simulink model "BLOQUEPSK"  (Simulink 8.4)
settings: Solver=ode45  StartTime=0.0  StopTime=0.01  RelTol=1e-3
libraries: commrandsrc2 x1, dspsigops x1
settings Model: Creator=Labcom  LastModifiedBy=mazo2

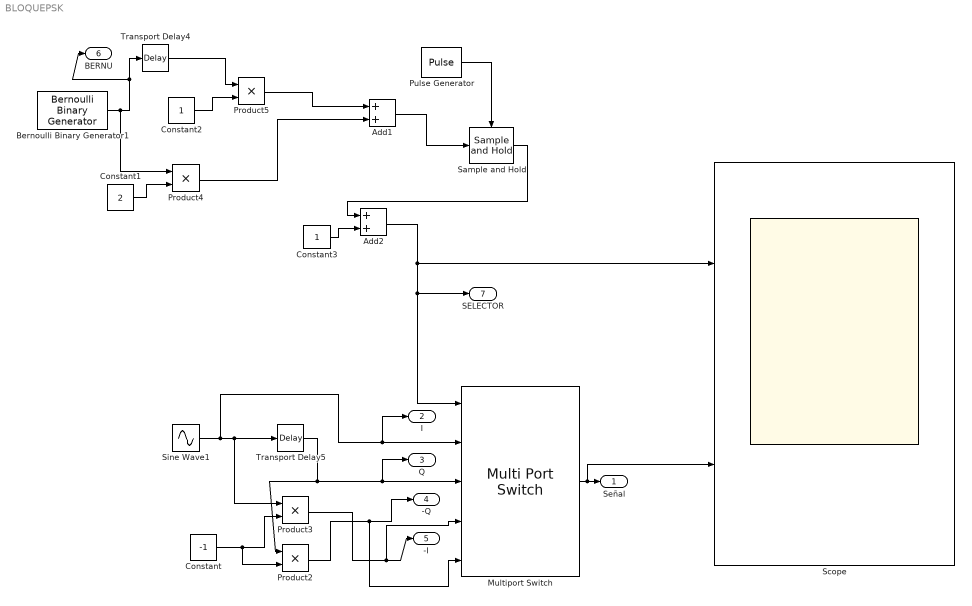
== system BLOQUEPSK ==
  Add1 : Sum
  Add2 : Sum
  Bernoulli Binary Generator1 : commrandsrc2/Bernoulli Binary Generator  P=0.5  seed=35  Ts=0.0005  frameBased=off  sampPerFrame=1  orient=off  outDataType=double
  Constant : Constant  Value=-1
  Constant1 : Constant  Value=2
  Constant2 : Constant
  Constant3 : Constant
  Multiport Switch : MultiPortSwitch  Inputs=4
  Product{2..5} (4 alike) : Product  RndMeth=Zero
  Pulse Generator : DiscretePulseGenerator  PulseType=Time based  Period=0.001  PulseWidth=90
  Sample and Hold : dspsigops/Sample and Hold  trig=Falling edge  initCond=0  latchinput=off
  Scope : Scope  NumInputPorts=2
      settings: TickLabels=on  TimeRange=0.01  YMin=-0~-1  YMax=4~1  MaxDataPoints=100000
  Sine Wave1 : Sin  Frequency=2*pi*1000000  SampleTime=0.00000001
  Transport Delay4 : TransportDelay  DelayTime=0.0005
  Transport Delay5 : TransportDelay  DelayTime=0.000001/4
  Señal : Outport
  I : Outport  Port=2
  Q : Outport  Port=3
  -Q : Outport  Port=4
  -I : Outport  Port=5
  BERNU : Outport  Port=6
  SELECTOR : Outport  Port=7
  wires:
  Sine Wave1/1 -> Transport Delay5/1, Product3/1, Multiport Switch/2, I/1
  Transport Delay5/1 -> Product2/1, Multiport Switch/3, Q/1
  Constant/1 -> Product3/2, Product2/2
  Bernoulli Binary Generator1/1 -> Product4/1, Transport Delay4/1, BERNU/1
  Product3/1 -> -I/1, Multiport Switch/4
  Product2/1 -> -Q/1, Multiport Switch/5
  Transport Delay4/1 -> Product5/1
  Constant1/1 -> Product4/2
  Constant2/1 -> Product5/2
  Product5/1 -> Add1/1
  Product4/1 -> Add1/2
  Constant3/1 -> Add2/2
  Add2/1 -> Multiport Switch/1, SELECTOR/1, Scope/1
  Multiport Switch/1 -> Señal/1, Scope/2
  Add1/1 -> Sample and Hold/1
  Sample and Hold/1 -> Add2/1
  Pulse Generator/1 -> Sample and Hold/Trigger
